simulink model "test_space"  (Simulink 8.9)
settings: Solver=VariableStepAuto  StartTime=0.0  StopTime=0.000001  RelTol=1e-3
libraries: dspxfrm3 x1, commsequence2 x1
settings Model: Creator=Alam  LastModifiedBy=Alam
settings Model: LogicAnalyzerGraphicalSettings=|
  | {
  |   "cursors" : {
  |     "activeCursor" : 0,
  |     "lockedCursors" : [
  | 
  |     ],
  |     "startingCursor" : 0,
  |     "times" : [
  |       0,
  |       0.0005130378096479791
  |     ]
  |   },
  |   "global" : {
  |     "format" : "digital",
  |     "groupCount" : 1,
  |     "radix" : "binary"
  |   },
  |   "panels" : [
  |     {
  |       "height" : 100,
  |       "startingTrace" : 0,
  |       "traces" : [
  | 
  |       ],
  |       "yOffset" : 0
  |     }
  |   ],
  |   "timeAxis" : {
  |     "displayUnits" : "u",
  |     "pixelsPerSecond" : 767000
  |   }
  | }
settings DataIOCC: LimitDataPoints=off  SaveFormat=Dataset  SignalLoggingSaveFormat=Dataset
settings OptimizationCC: LifeSpan=auto
settings DebuggingCC: UnderspecifiedInitializationDetection=Simplified  MergeDetectMultiDrivingBlocksExec=error  FcnCallInpInsideContextMsg=error  StateNameClashWarn=none  SFUnexpectedBacktrackingDiag=error  SFNoUnconditionalDefaultTransitionDiag=error  SFExecutionAtInitializationDiag=warning
settings HardwareCC: ProdBitPerPointer=64  ProdBitPerSizeT=64  ProdBitPerPtrDiffT=64  ProdLargestAtomicFloat=Float  ProdIntDivRoundTo=Zero  ProdEndianess=LittleEndian  ProdWordSize=64  ProdHWDeviceType=Intel->x86-64 (Windows64)
settings ModelReferenceCC: PropagateSignalLabelsOutOfModel=on
settings GRTTargetCC: TargetLangStandard=C99 (ISO)  GeneratePreprocessorConditionals=Use local settings  CombineOutputUpdateFcns=on  GRTInterface=off
settings ConfigComp: CovMetricSettings=dwe  CovHtmlReporting=off  CovSaveCumulativeToWorkspaceVar=off  CovSaveSingleToWorkspaceVar=off  CovExternalEMLEnable=on

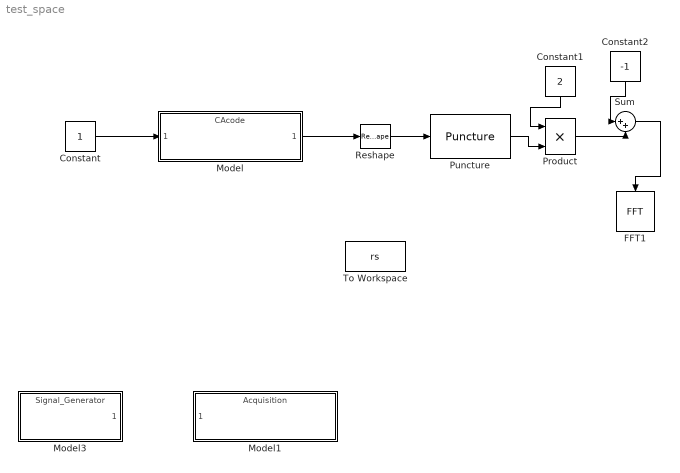
== system test_space ==
  Constant : Constant
  Constant1 : Constant  Value=2
  Constant2 : Constant  Value=-1
  FFT1 : dspxfrm3/FFT  FFTImplementation=Auto  CompMethod=Table lookup  TableOpt=NEW  TableOptActive=Speed  BitRevOrder=off  Normalize=off  InheritFFTLength=on  FFTLength=64  WrapInput=on  roundingMode=Floor  overflowMode=off  firstCoeffDataTypeStr=Inherit: Same word length as input  firstCoeffLastDataTypeStr=Inherit: Same word length as input  outputMin=[]  outputMax=[]
  Model : ModelReference  ModelNameDialog=CAcode.mdl  SimulationMode=Normal  ModelReferenceVersion=1.38
  Model1 : ModelReference  ModelNameDialog=Acquisition.mdl  SimulationMode=Normal  ModelReferenceVersion=1.42
  Model3 : ModelReference  ModelNameDialog=Signal_Generator.slx  SimulationMode=Normal  ModelReferenceVersion=1.6
  Product : Product
  Puncture : commsequence2/Puncture  punctureVector=[1;0]
      settings: SourceProductName=Communications System Toolbox  SourceProductBaseCode=CM
  Reshape : Reshape  OutputDimensionality=Column vector (2-D)
  Sum : Sum  Inputs=|++
  To Workspace : ToWorkspace  VariableName=rs  SampleTime=-1
  wires:
  Constant/1 -> Model/1
  Model/1 -> Reshape/1
  Reshape/1 -> Puncture/1
  Puncture/1 -> Product/2
  Product/1 -> Sum/2
  Constant1/1 -> Product/1
  Constant2/1 -> Sum/1
  Sum/1 -> FFT1/1
